simulink model "celab3"  (R2012b)
settings: Solver=ode45  StartTime=0.0  StopTime=10.0  RelTol=1e-3
settings Model: Creator=Krunal  LastModifiedBy=Krunal

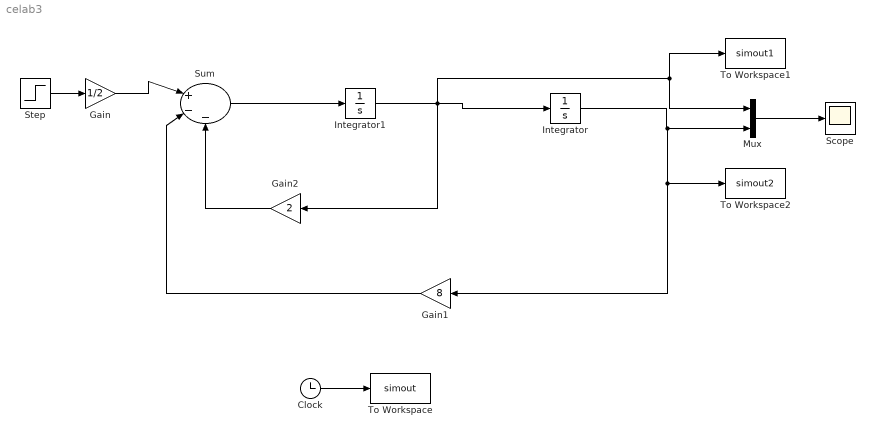
== system celab3 ==
  Clock : Clock
  Gain : Gain  Gain=1/2
  Gain1 : Gain  Gain=8
  Gain2 : Gain  Gain=2
  Integrator : Integrator
  Integrator1 : Integrator
  Mux : Mux  Inputs=2
  Scope : Scope
  Step : Step  SampleTime=0
  Sum : Sum  Inputs=|+--
  To Workspace : ToWorkspace  VariableName=simout  SampleTime=-1
  To Workspace1 : ToWorkspace  VariableName=simout1  SampleTime=-1
  To Workspace2 : ToWorkspace  VariableName=simout2  SampleTime=-1
  wires:
  Gain/1 -> Sum/1
  Sum/1 -> Integrator1/1
  Integrator1/1 -> Mux/1, To Workspace1/1, Gain2/1, Integrator/1
  Integrator/1 -> To Workspace2/1, Gain1/1, Mux/2
  Mux/1 -> Scope/1
  Gain2/1 -> Sum/3
  Gain1/1 -> Sum/2
  Step/1 -> Gain/1
  Clock/1 -> To Workspace/1
